simulink model "Colab_4Quad_model_01"  (R2018b)
settings: Solver=ode45  StartTime=0.0  StopTime=10  RelTol=1e-3
InitFcn:
  | Colab_4Quad_model_01_const
values from neighbouring files (symbols this model uses):
  All_rho = [d1 0 0 ... (first row only)    [Colab_4Quad_model_01_const.m]    (also in Colab_4Quad_model_02_const.m; Simple_4Quad_payload_04_const.m; Simple_4Quad_payload_05_const.m; Simple_4Quad_payload_06_const.m)
  d1 = 0.25    [Colab_4Quad_model_01_const.m]    (also in Colab_4Quad_model_02_const.m = 0.5; Simple_4Quad_payload_01_const.m = 1; Simple_4Quad_payload_02_const.m = 1; Simple_4Quad_payload_03_const.m = 1)
  d2 = 0.25    [Colab_4Quad_model_01_const.m]    (also in Colab_4Quad_model_02_const.m = 0.5; Simple_4Quad_payload_01_const.m = 1; Simple_4Quad_payload_02_const.m = 1; Simple_4Quad_payload_03_const.m = 1)
  g = 9.81    [Colab_4Quad_model_01_const.m]    (also in Colab_4Quad_model_02_const.m; Simple_2Quad_payload_01_const.m; Simple_2Quad_payload_02_const.m; Simple_2Quad_payload_03_const.m)
  Jo = diag([Ix;Iy;Iz])    [Colab_4Quad_model_01_const.m]    (also in Colab_4Quad_model_02_const.m; Simple_4Quad_payload_04_const.m; Simple_4Quad_payload_05_const.m; Simple_4Quad_payload_06_const.m)
  Jq = diag([0.0291 0.0291 0.0552])    [Colab_4Quad_model_01_const.m]    (also in Colab_4Quad_model_02_const.m = diag([0.03 0.03 0.06]); Simple_4Quad_payload_03_const.m = 1.2416e-3 * diag([1 1 2]); Simple_4Quad_payload_04_const.m = 1 * diag([1 1 2]); Simple_4Quad_payload_05_const.m = 1 * diag([1 1 2]))
  l = 3.1819    [Colab_4Quad_model_01_const.m]    (also in Colab_4Quad_model_02_const.m = 3; Simple_2Quad_payload_04_const.m = 1; Simple_4Quad_payload_01_const.m = 1; Simple_4Quad_payload_02_const.m = 2)
  M = 1.0    (= 1)    [Colab_4Quad_model_01_const.m]    (also in Colab_4Quad_model_02_const.m; Simple_2Quad_payload_01_const.m; Simple_2Quad_payload_02_const.m; Simple_2Quad_payload_03_const.m)
  m = 1.5    [Colab_4Quad_model_01_const.m]    (also in Colab_4Quad_model_02_const.m; Simple_2Quad_payload_04_const.m = 1; Simple_4Quad_payload_01_const.m = 1; Simple_4Quad_payload_02_const.m = 1)
  U0 = -20    [Colab_4Quad_model_01_const.m]    (also in Colab_4Quad_model_02_const.m)
settings Model: Creator=ali  LastModifiedBy=asafae
settings SolverCC: ZeroCrossAlgorithm=Adaptive
settings DebuggingCC: IgnoredZcDiagnostic=none

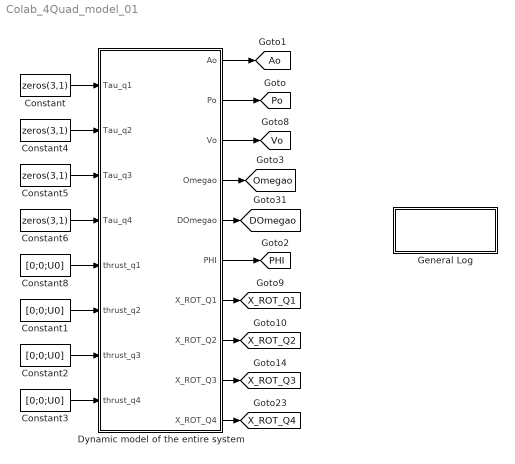
== system Colab_4Quad_model_01 ==
  Constant{,4..6} (4 alike) : Constant  Value=zeros(3,1)
  Constant{1..3,8} (4 alike) : Constant  Value=[0;0;U0]
  Dynamic model of the entire system : Subsystem
  General Log : Subsystem
  tag scope: Ao=global, DOmegao=global, Omegao=global, PHI=global, Po=global, Vo=global, X_ROT_Q1=global, X_ROT_Q2=global, X_ROT_Q3=global, X_ROT_Q4=global
  wires:
  Constant4/1 -> Dynamic model of the entire system/2(Tau_q2)
  Constant5/1 -> Dynamic model of the entire system/3(Tau_q3)
  Constant6/1 -> Dynamic model of the entire system/4(Tau_q4)
  Dynamic model of the entire system/6(PHI) -> [PHI]
  Dynamic model of the entire system/4(Omegao) -> [Omegao]
  Dynamic model of the entire system/1(Ao) -> [Ao]
  Dynamic model of the entire system/2(Po) -> [Po]
  Dynamic model of the entire system/5(DOmegao) -> [DOmegao]
  Dynamic model of the entire system/7(X_ROT_Q1) -> [X_ROT_Q1]
  Dynamic model of the entire system/8(X_ROT_Q2) -> [X_ROT_Q2]
  Dynamic model of the entire system/9(X_ROT_Q3) -> [X_ROT_Q3]
  Dynamic model of the entire system/3(Vo) -> [Vo]
  Dynamic model of the entire system/10(X_ROT_Q4) -> [X_ROT_Q4]
  Constant/1 -> Dynamic model of the entire system/1(Tau_q1)
  Constant8/1 -> Dynamic model of the entire system/5(thrust_q1)
  Constant1/1 -> Dynamic model of the entire system/6(thrust_q2)
  Constant2/1 -> Dynamic model of the entire system/7(thrust_q3)
  Constant3/1 -> Dynamic model of the entire system/8(thrust_q4)

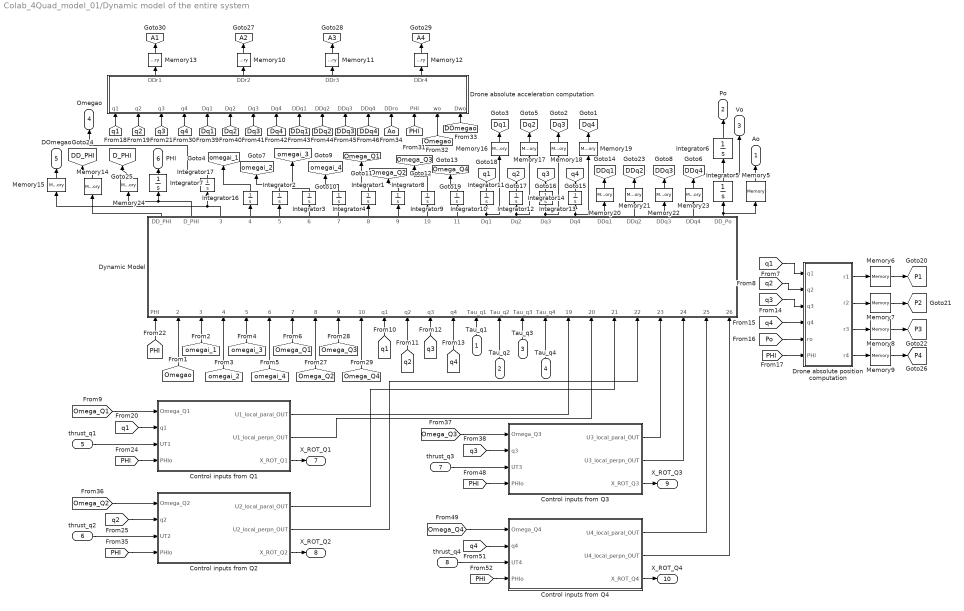
== system Colab_4Quad_model_01/Dynamic model of the entire system ==
  Tau_q1 : Inport
  Tau_q2 : Inport  Port=2
  Tau_q3 : Inport  Port=3
  Tau_q4 : Inport  Port=4
  thrust_q1 : Inport  Port=5
  thrust_q2 : Inport  Port=6
  thrust_q3 : Inport  Port=7
  thrust_q4 : Inport  Port=8
  Control inputs from Q1 : Subsystem
  Control inputs from Q2 : Subsystem
  Control inputs from Q3 : Subsystem
  Control inputs from Q4 : Subsystem
  Drone absolute acceleration computation : MATLAB Function  TreatAsAtomicUnit=on
  Drone absolute position computation : MATLAB Function  TreatAsAtomicUnit=on
  "Dynamic Model " : MATLAB Function  TreatAsAtomicUnit=on
  Integrator{1..5,7..10,16..17} (11 alike) : Integrator  InitialCondition=zeros(3,1)
  Integrator{11..14} (4 alike) : Integrator  InitialCondition=[0;0;1]
  Integrator6 : Integrator  InitialCondition=[0;0;0]
  Memory{5,10..24} (16 alike) : Memory  InitialCondition=zeros(3,1)
  Memory6 : Memory  InitialCondition=[d1;0;l]
  Memory7 : Memory  InitialCondition=[-d1;0;l]
  Memory8 : Memory  InitialCondition=[0;d2;l]
  Memory9 : Memory  InitialCondition=[0;-d2;l]
  Ao : Outport
  Po : Outport  Port=2
  Vo : Outport  Port=3
  Omegao : Outport  Port=4
  DOmegao : Outport  Port=5
  PHI : Outport  Port=6
  X_ROT_Q1 : Outport  Port=7
  X_ROT_Q2 : Outport  Port=8
  X_ROT_Q3 : Outport  Port=9
  X_ROT_Q4 : Outport  Port=10
  tag scope: A1=global, A2=global, A3=global, A4=global, DD_PHI=global, DDq1=global, DDq2=global, DDq3=global, DDq4=global, D_PHI=global, Dq1=global, Dq2=global, Dq3=global, Dq4=global, Omega_Q1=global, Omega_Q2=global, Omega_Q3=global, Omega_Q4=global, P1=global, P2=global, P3=global, P4=global, omegai_1=global, omegai_2=global, omegai_3=global, omegai_4=global, q1=global, q2=global, q3=global, q4=global
  wires:
  Integrator5/1 -> Vo/1, Integrator6/1
  Integrator1/1 -> [Omega_Q1]
  Integrator2/1 -> [omegai_2]
  Integrator3/1 -> [omegai_3]
  Integrator6/1 -> Po/1
  Integrator4/1 -> [omegai_4]
  Memory5/1 -> Ao/1
  Integrator7/1 -> PHI/1
  "Dynamic Model "/20(DD_Po) -> Memory5/1, Integrator5/1
  "Dynamic Model "/2(D_PHI) -> Memory24/1, Integrator7/1
  "Dynamic Model "/1(DD_PHI) -> Memory14/1
  "Dynamic Model "/7(D_omegai_4) -> Integrator4/1
  "Dynamic Model "/6(D_omegai_3) -> Integrator3/1
  "Dynamic Model "/5(D_omegai_2) -> Integrator2/1
  "Dynamic Model "/4(D_omegai_1) -> Integrator16/1
  "Dynamic Model "/3(D_Omegao) -> Memory15/1, Integrator17/1
  Integrator16/1 -> [omegai_1]
  "Dynamic Model "/8(D_Omega_Q1) -> Integrator1/1
  "Dynamic Model "/9(D_Omega_Q2) -> Integrator8/1
  "Dynamic Model "/10(D_Omega_Q3) -> Integrator9/1
  "Dynamic Model "/11(D_Omega_Q4) -> Integrator10/1
  Integrator8/1 -> [Omega_Q2]
  Integrator10/1 -> [Omega_Q4]
  Integrator9/1 -> [Omega_Q3]
  "Dynamic Model "/12(Dq1) -> Memory16/1, Integrator11/1
  "Dynamic Model "/13(Dq2) -> Memory17/1, Integrator12/1
  "Dynamic Model "/14(Dq3) -> Memory18/1, Integrator13/1
  "Dynamic Model "/15(Dq4) -> Memory19/1, Integrator14/1
  Integrator14/1 -> [q4]
  Integrator13/1 -> [q3]
  Integrator12/1 -> [q2]
  Integrator11/1 -> [q1]
  [PHI] -> "Dynamic Model "/1(PHI)
  [Omegao] -> "Dynamic Model "/2(Omegao)
  [omegai_1] -> "Dynamic Model "/3(omegai1)
  [omegai_2] -> "Dynamic Model "/4(omegai2)
  [omegai_3] -> "Dynamic Model "/5(omegai3)
  [omegai_4] -> "Dynamic Model "/6(omegai4)
  [Omega_Q1] -> "Dynamic Model "/7(Omega_q1)
  [Omega_Q2] -> "Dynamic Model "/8(Omega_q2)
  [Omega_Q3] -> "Dynamic Model "/9(Omega_q3)
  [Omega_Q4] -> "Dynamic Model "/10(Omega_q4)
  [q1] -> "Dynamic Model "/11(q1)
  [q2] -> "Dynamic Model "/12(q2)
  [q3] -> "Dynamic Model "/13(q3)
  [q4] -> "Dynamic Model "/14(q4)
  Tau_q2/1 -> "Dynamic Model "/16(Tau_q2)
  Tau_q4/1 -> "Dynamic Model "/18(Tau_q4)
  Tau_q1/1 -> "Dynamic Model "/15(Tau_q1)
  Tau_q3/1 -> "Dynamic Model "/17(Tau_q3)
  Control inputs from Q1/1(U1_local_paral_OUT) -> "Dynamic Model "/19(U1_local_paral)
  [q1] -> Drone absolute position computation/1(q1)
  [q2] -> Drone absolute position computation/2(q2)
  [q3] -> Drone absolute position computation/3(q3)
  [q4] -> Drone absolute position computation/4(q4)
  [Po] -> Drone absolute position computation/5(ro)
  [PHI] -> Drone absolute position computation/6(PHI)
  Memory6/1 -> [P1]
  Memory8/1 -> [P3]
  Memory7/1 -> [P2]
  Memory9/1 -> [P4]
  Drone absolute position computation/4(r4) -> Memory9/1
  Drone absolute position computation/3(r3) -> Memory8/1
  Drone absolute position computation/2(r2) -> Memory7/1
  Drone absolute position computation/1(r1) -> Memory6/1
  [q1] -> Drone absolute acceleration computation/1(q1)
  [q2] -> Drone absolute acceleration computation/2(q2)
  [q3] -> Drone absolute acceleration computation/3(q3)
  [q4] -> Drone absolute acceleration computation/4(q4)
  [PHI] -> Drone absolute acceleration computation/14(PHI)
  [Omegao] -> Drone absolute acceleration computation/15(wo)
  Memory13/1 -> [A1]
  Drone absolute acceleration computation/1(DDr1) -> Memory13/1
  Memory10/1 -> [A2]
  Drone absolute acceleration computation/2(DDr2) -> Memory10/1
  Memory11/1 -> [A3]
  Drone absolute acceleration computation/3(DDr3) -> Memory11/1
  Memory12/1 -> [A4]
  Drone absolute acceleration computation/4(DDr4) -> Memory12/1
  Memory15/1 -> DOmegao/1
  [DOmegao] -> Drone absolute acceleration computation/16(Dwo)
  [Ao] -> Drone absolute acceleration computation/13(DDro)
  Memory19/1 -> [Dq4]
  Memory18/1 -> [Dq3]
  Memory16/1 -> [Dq1]
  Memory17/1 -> [Dq2]
  [Dq4] -> Drone absolute acceleration computation/8(Dq4)
  [Dq3] -> Drone absolute acceleration computation/7(Dq3)
  [Dq2] -> Drone absolute acceleration computation/6(Dq2)
  [Dq1] -> Drone absolute acceleration computation/5(Dq1)
  Memory21/1 -> [DDq2]
  Memory20/1 -> [DDq1]
  Memory22/1 -> [DDq3]
  Memory23/1 -> [DDq4]
  "Dynamic Model "/16(DDq1) -> Memory20/1
  "Dynamic Model "/17(DDq2) -> Memory21/1
  "Dynamic Model "/18(DDq3) -> Memory22/1
  "Dynamic Model "/19(DDq4) -> Memory23/1
  [DDq1] -> Drone absolute acceleration computation/9(DDq1)
  [DDq2] -> Drone absolute acceleration computation/10(DDq2)
  [DDq3] -> Drone absolute acceleration computation/11(DDq3)
  [DDq4] -> Drone absolute acceleration computation/12(DDq4)
  Memory24/1 -> [D_PHI]
  Control inputs from Q3/1(U3_local_paral_OUT) -> "Dynamic Model "/23(U3_local_paral)
  Control inputs from Q4/1(U4_local_paral_OUT) -> "Dynamic Model "/25(U4_local_paral)
  Control inputs from Q4/2(U4_local_perpn_OUT) -> "Dynamic Model "/26(U4_local_perpn)
  Control inputs from Q1/3(X_ROT_Q1) -> X_ROT_Q1/1
  [Omega_Q1] -> Control inputs from Q1/1(Omega_Q1)
  Control inputs from Q1/2(U1_local_perpn_OUT) -> "Dynamic Model "/20(U1_local_perpn)
  [q1] -> Control inputs from Q1/2(q1)
  thrust_q1/1 -> Control inputs from Q1/3(UT1)
  [PHI] -> Control inputs from Q1/4(PHIo)
  [PHI] -> Control inputs from Q2/4(PHIo)
  thrust_q2/1 -> Control inputs from Q2/3(UT2)
  [q2] -> Control inputs from Q2/2(q2)
  [Omega_Q2] -> Control inputs from Q2/1(Omega_Q2)
  Control inputs from Q2/3(X_ROT_Q2) -> X_ROT_Q2/1
  Control inputs from Q2/1(U2_local_paral_OUT) -> "Dynamic Model "/21(U2_local_paral)
  Control inputs from Q2/2(U2_local_perpn_OUT) -> "Dynamic Model "/22(U2_local_perpn)
  [Omega_Q3] -> Control inputs from Q3/1(Omega_Q3)
  Control inputs from Q3/3(X_ROT_Q3) -> X_ROT_Q3/1
  Control inputs from Q3/2(U3_local_perpn_OUT) -> "Dynamic Model "/24(U3_local_perpn)
  [q3] -> Control inputs from Q3/2(q3)
  [PHI] -> Control inputs from Q3/4(PHIo)
  Control inputs from Q4/3(X_ROT_Q4) -> X_ROT_Q4/1
  [Omega_Q4] -> Control inputs from Q4/1(Omega_Q4)
  [q4] -> Control inputs from Q4/2(q4)
  [PHI] -> Control inputs from Q4/4(PHIo)
  Memory14/1 -> [DD_PHI]
  thrust_q4/1 -> Control inputs from Q4/3(UT4)
  Integrator17/1 -> Omegao/1
  thrust_q3/1 -> Control inputs from Q3/3(UT3)

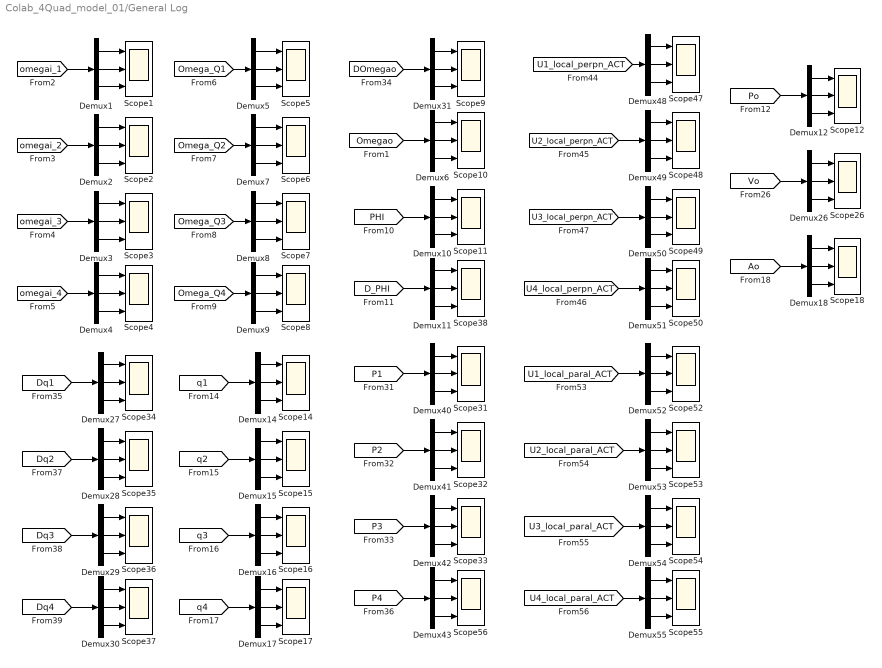
== system Colab_4Quad_model_01/General Log ==
  Demux{1..12,14..18,26..31,40..43,48..55} (35 alike) : Demux  Outputs=3
  Scope{1..12,14..18,26,31..38,47..50,52..56} (35 alike) : Scope  NumInputPorts=3
  wires:
  Demux6/2 -> Scope10/2
  Demux6/1 -> Scope10/1
  Demux6/3 -> Scope10/3
  [Omegao] -> Demux6/1
  [omegai_1] -> Demux1/1
  Demux1/3 -> Scope1/3
  Demux1/1 -> Scope1/1
  Demux1/2 -> Scope1/2
  Demux2/2 -> Scope2/2
  Demux2/1 -> Scope2/1
  Demux2/3 -> Scope2/3
  [omegai_2] -> Demux2/1
  [omegai_3] -> Demux3/1
  Demux3/3 -> Scope3/3
  Demux3/1 -> Scope3/1
  Demux3/2 -> Scope3/2
  Demux4/2 -> Scope4/2
  Demux4/1 -> Scope4/1
  Demux4/3 -> Scope4/3
  [omegai_4] -> Demux4/1
  [Omega_Q4] -> Demux9/1
  Demux9/3 -> Scope8/3
  Demux9/1 -> Scope8/1
  Demux9/2 -> Scope8/2
  Demux8/2 -> Scope7/2
  Demux8/1 -> Scope7/1
  Demux8/3 -> Scope7/3
  [Omega_Q3] -> Demux8/1
  [Omega_Q2] -> Demux7/1
  Demux7/3 -> Scope6/3
  Demux7/1 -> Scope6/1
  Demux7/2 -> Scope6/2
  Demux5/2 -> Scope5/2
  Demux5/1 -> Scope5/1
  Demux5/3 -> Scope5/3
  [Omega_Q1] -> Demux5/1
  [PHI] -> Demux10/1
  Demux10/3 -> Scope11/3
  Demux10/1 -> Scope11/1
  Demux10/2 -> Scope11/2
  Demux11/2 -> Scope38/2
  Demux11/1 -> Scope38/1
  Demux11/3 -> Scope38/3
  [D_PHI] -> Demux11/1
  [Po] -> Demux12/1
  Demux12/3 -> Scope12/3
  Demux12/1 -> Scope12/1
  Demux12/2 -> Scope12/2
  [q4] -> Demux17/1
  Demux17/3 -> Scope17/3
  Demux17/1 -> Scope17/1
  Demux17/2 -> Scope17/2
  Demux16/2 -> Scope16/2
  Demux16/1 -> Scope16/1
  Demux16/3 -> Scope16/3
  [q3] -> Demux16/1
  [q2] -> Demux15/1
  Demux15/3 -> Scope15/3
  Demux15/1 -> Scope15/1
  Demux15/2 -> Scope15/2
  Demux14/2 -> Scope14/2
  Demux14/1 -> Scope14/1
  Demux14/3 -> Scope14/3
  [q1] -> Demux14/1
  [Vo] -> Demux26/1
  Demux26/3 -> Scope26/3
  Demux26/1 -> Scope26/1
  Demux26/2 -> Scope26/2
  [DOmegao] -> Demux31/1
  Demux31/3 -> Scope9/3
  Demux31/1 -> Scope9/1
  Demux31/2 -> Scope9/2
  [Dq1] -> Demux27/1
  Demux27/3 -> Scope34/3
  Demux27/1 -> Scope34/1
  Demux27/2 -> Scope34/2
  Demux28/2 -> Scope35/2
  Demux28/1 -> Scope35/1
  Demux28/3 -> Scope35/3
  [Dq2] -> Demux28/1
  [Dq3] -> Demux29/1
  Demux29/3 -> Scope36/3
  Demux29/1 -> Scope36/1
  Demux29/2 -> Scope36/2
  Demux30/2 -> Scope37/2
  Demux30/1 -> Scope37/1
  Demux30/3 -> Scope37/3
  [Dq4] -> Demux30/1
  [P1] -> Demux40/1
  Demux40/3 -> Scope31/3
  Demux40/2 -> Scope31/2
  Demux41/2 -> Scope32/2
  Demux41/1 -> Scope32/1
  Demux41/3 -> Scope32/3
  [P2] -> Demux41/1
  [P3] -> Demux42/1
  Demux42/3 -> Scope33/3
  Demux42/1 -> Scope33/1
  Demux42/2 -> Scope33/2
  Demux43/2 -> Scope56/2
  Demux43/1 -> Scope56/1
  Demux43/3 -> Scope56/3
  [P4] -> Demux43/1
  Demux40/1 -> Scope31/1
  [U2_local_paral_ACT] -> Demux53/1
  [U3_local_paral_ACT] -> Demux54/1
  [U4_local_paral_ACT] -> Demux55/1
  [U1_local_paral_ACT] -> Demux52/1
  Demux52/3 -> Scope52/3
  Demux52/1 -> Scope52/1
  Demux52/2 -> Scope52/2
  Demux53/2 -> Scope53/2
  Demux53/1 -> Scope53/1
  Demux53/3 -> Scope53/3
  Demux54/3 -> Scope54/3
  Demux54/1 -> Scope54/1
  Demux54/2 -> Scope54/2
  Demux55/2 -> Scope55/2
  Demux55/1 -> Scope55/1
  Demux55/3 -> Scope55/3
  [U4_local_perpn_ACT] -> Demux51/1
  Demux51/3 -> Scope50/3
  Demux51/1 -> Scope50/1
  Demux51/2 -> Scope50/2
  Demux50/2 -> Scope49/2
  Demux50/1 -> Scope49/1
  Demux50/3 -> Scope49/3
  [U3_local_perpn_ACT] -> Demux50/1
  [U2_local_perpn_ACT] -> Demux49/1
  Demux49/3 -> Scope48/3
  Demux49/1 -> Scope48/1
  Demux49/2 -> Scope48/2
  Demux48/2 -> Scope47/2
  Demux48/1 -> Scope47/1
  Demux48/3 -> Scope47/3
  [U1_local_perpn_ACT] -> Demux48/1
  [Ao] -> Demux18/1
  Demux18/3 -> Scope18/3
  Demux18/1 -> Scope18/1
  Demux18/2 -> Scope18/2

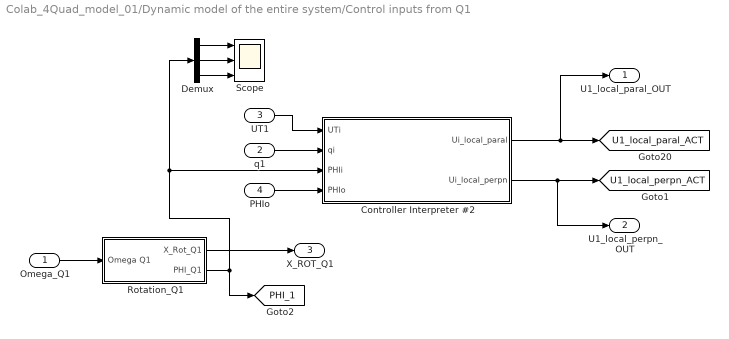
== system Colab_4Quad_model_01/Dynamic model of the entire system/Control inputs from Q1 ==
  Omega_Q1 : Inport
  q1 : Inport  Port=2
  UT1 : Inport  Port=3
  PHIo : Inport  Port=4
  Controller Interpreter #2 : MATLAB Function  TreatAsAtomicUnit=on
  Demux : Demux  Outputs=3
  Rotation_Q1 : Subsystem
  Scope : Scope  NumInputPorts=3
  U1_local_paral_OUT : Outport
  U1_local_perpn_OUT : Outport  Port=2
  X_ROT_Q1 : Outport  Port=3
  tag scope: PHI_1=global, U1_local_paral_ACT=global, U1_local_perpn_ACT=global
  wires:
  UT1/1 -> Controller Interpreter #2/1(UTi)
  q1/1 -> Controller Interpreter #2/2(qi)
  Omega_Q1/1 -> Rotation_Q1/1(Omega Q1)
  Rotation_Q1/1(X_Rot_Q1) -> X_ROT_Q1/1
  PHIo/1 -> Controller Interpreter #2/4(PHIo)
  Controller Interpreter #2/2(Ui_local_perpn) -> U1_local_perpn_OUT/1, [U1_local_perpn_ACT]
  Controller Interpreter #2/1(Ui_local_paral) -> U1_local_paral_OUT/1, [U1_local_paral_ACT]
  Demux/1 -> Scope/1
  Demux/2 -> Scope/2
  Demux/3 -> Scope/3
  Rotation_Q1/2(PHI_Q1) -> [PHI_1], Controller Interpreter #2/3(PHIi), Demux/1

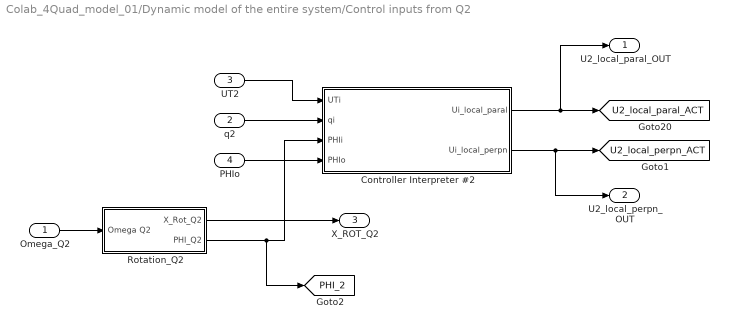
== system Colab_4Quad_model_01/Dynamic model of the entire system/Control inputs from Q2 ==
  Omega_Q2 : Inport
  q2 : Inport  Port=2
  UT2 : Inport  Port=3
  PHIo : Inport  Port=4
  Controller Interpreter #2 : MATLAB Function  TreatAsAtomicUnit=on
  Rotation_Q2 : Subsystem
  U2_local_paral_OUT : Outport
  U2_local_perpn_OUT : Outport  Port=2
  X_ROT_Q2 : Outport  Port=3
  tag scope: PHI_2=global, U2_local_paral_ACT=global, U2_local_perpn_ACT=global
  wires:
  PHIo/1 -> Controller Interpreter #2/4(PHIo)
  Rotation_Q2/1(X_Rot_Q2) -> X_ROT_Q2/1
  Omega_Q2/1 -> Rotation_Q2/1(Omega Q2)
  q2/1 -> Controller Interpreter #2/2(qi)
  UT2/1 -> Controller Interpreter #2/1(UTi)
  Controller Interpreter #2/2(Ui_local_perpn) -> U2_local_perpn_OUT/1, [U2_local_perpn_ACT]
  Controller Interpreter #2/1(Ui_local_paral) -> U2_local_paral_OUT/1, [U2_local_paral_ACT]
  Rotation_Q2/2(PHI_Q2) -> [PHI_2], Controller Interpreter #2/3(PHIi)

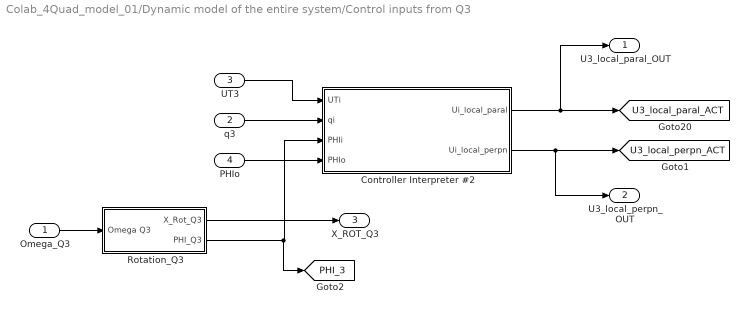
== system Colab_4Quad_model_01/Dynamic model of the entire system/Control inputs from Q3 ==
  Omega_Q3 : Inport
  q3 : Inport  Port=2
  UT3 : Inport  Port=3
  PHIo : Inport  Port=4
  Controller Interpreter #2 : MATLAB Function  TreatAsAtomicUnit=on
  Rotation_Q3 : Subsystem
  U3_local_paral_OUT : Outport
  U3_local_perpn_OUT : Outport  Port=2
  X_ROT_Q3 : Outport  Port=3
  tag scope: PHI_3=global, U3_local_paral_ACT=global, U3_local_perpn_ACT=global
  wires:
  UT3/1 -> Controller Interpreter #2/1(UTi)
  q3/1 -> Controller Interpreter #2/2(qi)
  Omega_Q3/1 -> Rotation_Q3/1(Omega Q3)
  Rotation_Q3/1(X_Rot_Q3) -> X_ROT_Q3/1
  PHIo/1 -> Controller Interpreter #2/4(PHIo)
  Controller Interpreter #2/2(Ui_local_perpn) -> U3_local_perpn_OUT/1, [U3_local_perpn_ACT]
  Controller Interpreter #2/1(Ui_local_paral) -> U3_local_paral_OUT/1, [U3_local_paral_ACT]
  Rotation_Q3/2(PHI_Q3) -> [PHI_3], Controller Interpreter #2/3(PHIi)

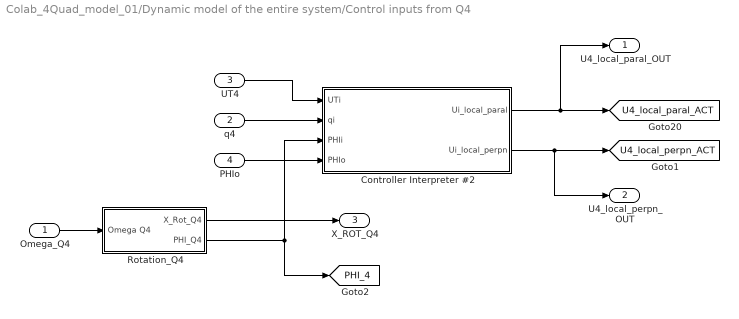
== system Colab_4Quad_model_01/Dynamic model of the entire system/Control inputs from Q4 ==
  Omega_Q4 : Inport
  q4 : Inport  Port=2
  UT4 : Inport  Port=3
  PHIo : Inport  Port=4
  Controller Interpreter #2 : MATLAB Function  TreatAsAtomicUnit=on
  Rotation_Q4 : Subsystem
  U4_local_paral_OUT : Outport
  U4_local_perpn_OUT : Outport  Port=2
  X_ROT_Q4 : Outport  Port=3
  tag scope: PHI_4=global, U4_local_paral_ACT=global, U4_local_perpn_ACT=global
  wires:
  PHIo/1 -> Controller Interpreter #2/4(PHIo)
  Rotation_Q4/1(X_Rot_Q4) -> X_ROT_Q4/1
  Omega_Q4/1 -> Rotation_Q4/1(Omega Q4)
  q4/1 -> Controller Interpreter #2/2(qi)
  UT4/1 -> Controller Interpreter #2/1(UTi)
  Controller Interpreter #2/1(Ui_local_paral) -> U4_local_paral_OUT/1, [U4_local_paral_ACT]
  Rotation_Q4/2(PHI_Q4) -> Controller Interpreter #2/3(PHIi), [PHI_4]
  Controller Interpreter #2/2(Ui_local_perpn) -> U4_local_perpn_OUT/1, [U4_local_perpn_ACT]

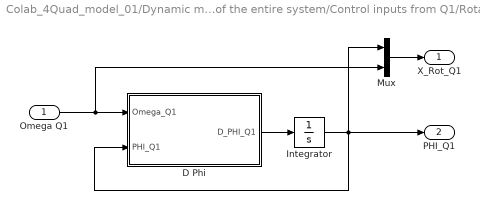
== system Colab_4Quad_model_01/Dynamic model of the entire system/Control inputs from Q1/Rotation_Q1 ==
  Omega Q1 : Inport
  D Phi : MATLAB Function  TreatAsAtomicUnit=on
  Integrator : Integrator  InitialCondition=zeros(3,1)
  Mux : Mux  Inputs=2
  X_Rot_Q1 : Outport
  PHI_Q1 : Outport  Port=2
  wires:
  D Phi/1(D_PHI_Q1) -> Integrator/1
  Omega Q1/1 -> D Phi/1(Omega_Q1), Mux/2
  Integrator/1 -> PHI_Q1/1, D Phi/2(PHI_Q1), Mux/1
  Mux/1 -> X_Rot_Q1/1

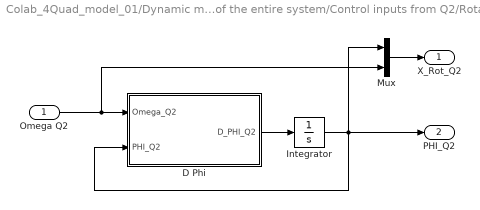
== system Colab_4Quad_model_01/Dynamic model of the entire system/Control inputs from Q2/Rotation_Q2 ==
  Omega Q2 : Inport
  D Phi : MATLAB Function  TreatAsAtomicUnit=on
  Integrator : Integrator  InitialCondition=zeros(3,1)
  Mux : Mux  Inputs=2
  X_Rot_Q2 : Outport
  PHI_Q2 : Outport  Port=2
  wires:
  D Phi/1(D_PHI_Q2) -> Integrator/1
  Omega Q2/1 -> Mux/2, D Phi/1(Omega_Q2)
  Integrator/1 -> PHI_Q2/1, D Phi/2(PHI_Q2), Mux/1
  Mux/1 -> X_Rot_Q2/1

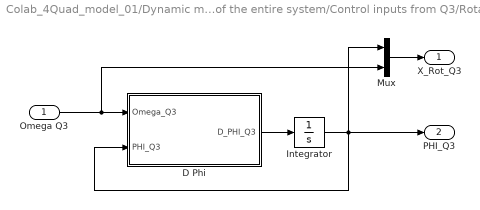
== system Colab_4Quad_model_01/Dynamic model of the entire system/Control inputs from Q3/Rotation_Q3 ==
  Omega Q3 : Inport
  D Phi : MATLAB Function  TreatAsAtomicUnit=on
  Integrator : Integrator  InitialCondition=zeros(3,1)
  Mux : Mux  Inputs=2
  X_Rot_Q3 : Outport
  PHI_Q3 : Outport  Port=2
  wires:
  D Phi/1(D_PHI_Q3) -> Integrator/1
  Omega Q3/1 -> Mux/2, D Phi/1(Omega_Q3)
  Integrator/1 -> PHI_Q3/1, D Phi/2(PHI_Q3), Mux/1
  Mux/1 -> X_Rot_Q3/1

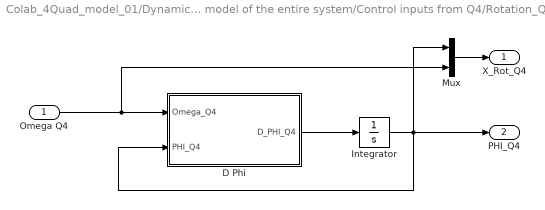
== system Colab_4Quad_model_01/Dynamic model of the entire system/Control inputs from Q4/Rotation_Q4 ==
  Omega Q4 : Inport
  D Phi : MATLAB Function  TreatAsAtomicUnit=on
  Integrator : Integrator  InitialCondition=zeros(3,1)
  Mux : Mux  Inputs=2
  X_Rot_Q4 : Outport
  PHI_Q4 : Outport  Port=2
  wires:
  D Phi/1(D_PHI_Q4) -> Integrator/1
  Integrator/1 -> PHI_Q4/1, D Phi/2(PHI_Q4), Mux/1
  Mux/1 -> X_Rot_Q4/1
  Omega Q4/1 -> D Phi/1(Omega_Q4), Mux/2

== matlab function Colab_4Quad_model_01/Dynamic model of the entire system/Control inputs from Q1/Rotation_Q1/D Phi ==
  data: Omega_Q1 input; D_PHI_Q1 output; PHI_Q1 input
function D_PHI_Q1 = fcn(Omega_Q1,PHI_Q1)

phi_q1 = PHI_Q1(1);
theta_q1 = PHI_Q1(2);

Rm_Q1 = [1 0 -sin(theta_q1);
    0 cos(phi_q1) cos(theta_q1)*sin(phi_q1);
    0 -sin(phi_q1) cos(theta_q1)*cos(phi_q1)];

D_PHI_Q1 = (Rm_Q1)^(-1) * Omega_Q1;


end

== matlab function Colab_4Quad_model_01/Dynamic model of the entire system/Dynamic Model  ==
  data: DD_PHI output; D_PHI output; D_Omegao output; D_omegai_1 output; D_omegai_2 output; D_omegai_3 output; D_omegai_4 output; D_Omega_Q1 output; D_Omega_Q2 output; D_Omega_Q3 output; D_Omega_Q4 output; Dq1 output; Dq2 output; Dq3 output; Dq4 output; DDq1 output; DDq2 output; DDq3 output; DDq4 output; PHI input; Omegao input; omegai1 input; omegai2 input; omegai3 input; omegai4 input; Omega_q1 input; Omega_q2 input; Omega_q3 input; Omega_q4 input; q1 input; q2 input; q3 input; q4 input; DD_Po output; M parameter; Jo parameter; g parameter; m parameter; l parameter; Tau_q1 input; Tau_q2 input; Tau_q3 input; Tau_q4 input; Jq parameter; U1_local_paral input; U1_local_perpn input; U2_local_paral input; U2_local_perpn input; U3_local_paral input; U3_local_perpn input; U4_local_paral input; U4_local_perpn input; All_rho parameter
function [DD_PHI,D_PHI,D_Omegao,D_omegai_1,D_omegai_2,D_omegai_3,D_omegai_4,D_Omega_Q1,D_Omega_Q2,D_Omega_Q3,D_Omega_Q4,Dq1,Dq2,Dq3,Dq4,DDq1,DDq2,DDq3,DDq4,DD_Po] = ...
    fcn(PHI,Omegao,omegai1,omegai2,omegai3,omegai4,Omega_q1,Omega_q2,Omega_q3,Omega_q4,q1,q2,q3,q4,M,Jo,g,m, l,Tau_q1,Tau_q2,Tau_q3,Tau_q4, Jq, U1_local_paral,U1_local_perpn,U2_local_paral,U2_local_perpn,...
    U3_local_paral,U3_local_perpn,U4_local_paral,U4_local_perpn, All_rho)

phi = PHI(1);
theta = PHI(2);
psi = PHI(3);

Ro = [cos(psi)*cos(theta) cos(psi)*sin(theta)*sin(phi)-sin(psi)*cos(phi) cos(psi)*sin(theta)*cos(phi)+sin(psi)*sin(phi);
    sin(psi)*cos(theta) sin(psi)*sin(theta)*sin(phi)+cos(psi)*cos(phi) sin(psi)*sin(theta)*cos(phi)-cos(psi)*sin(phi);
    -sin(theta) cos(theta)*sin(phi) cos(theta)*cos(phi)];

r1 = All_rho(1,:)';
r2 = All_rho(2,:)';
r3 = All_rho(3,:)';
r4 = All_rho(4,:)';

G = [0;0;-g];

%% 
Ui_local_paral = struct('val',repmat({zeros(3,1)},4,1));
Ui_local_perpn = struct('val',repmat({zeros(3,1)},4,1));
ri = struct('val',repmat({zeros(3,1)},4,1));
ri_skew = struct('val',repmat({zeros(3)},4,1));
qi_body = struct('val',repmat({zeros(3,1)},4,1));
qi_inert = struct('val',repmat({zeros(3,1)},4,1));
qi_inert_skew = struct('val',repmat({zeros(3)},4,1));
Mq = struct('val',repmat({zeros(3,1)},4,1));
Omega_Qi_skew = struct('val',repmat({zeros(3)},4,1));
Omega_Qi = struct('val',repmat({zeros(3,1)},4,1));
D_Omega_Qi = struct('val',repmat({zeros(3,1)},4,1));

Ui_local_paral(1).val = U1_local_paral;
Ui_local_paral(2).val = U2_local_paral;
Ui_local_paral(3).val = U3_local_paral;
Ui_local_paral(4).val = U4_local_paral;

Ui_local_perpn(1).val = U1_local_perpn;
Ui_local_perpn(2).val = U2_local_perpn;
Ui_local_perpn(3).val = U3_local_perpn;
Ui_local_perpn(4).val = U4_local_perpn;

ri(1).val = r1;
ri(2).val = r2;
ri(3).val = r3;
ri(4).val = r4;

ri_skew(1).val = ... 
    [0 -r1(3) r1(2);
    r1(3) 0 -r1(1);
    -r1(2) r1(1) 0];

ri_skew(2).val = ... 
    [0 -r2(3) r2(2);
    r2(3) 0 -r2(1);
    -r2(2) r2(1) 0];

ri_skew(3).val = ... 
    [0 -r3(3) r3(2);
    r3(3) 0 -r3(1);
    -r3(2) r3(1) 0];

ri_skew(4).val = ... 
    [0 -r4(3) r4(2);
    r4(3) 0 -r4(1);
    -r4(2) r4(1) 0];

qi_body(1).val = -[q1(1);q1(2);q1(3)];
qi_body(2).val = -[q2(1);q2(2);q2(3)];
qi_body(3).val = -[q3(1);q3(2);q3(3)];
qi_body(4).val = -[q4(1);q4(2);q4(3)];

qi_inert(1).val = Ro * qi_body(1).val;
qi_inert(2).val = Ro * qi_body(2).val;
qi_inert(3).val = Ro * qi_body(3).val;
qi_inert(4).val = Ro * qi_body(4).val;

qi_inert_skew(1).val = ...
    [0 -qi_inert(1).val(3) qi_inert(1).val(2);
    qi_inert(1).val(3) 0 -qi_inert(1).val(1);
    -qi_inert(1).val(2) qi_inert(1).val(1) 0];

qi_inert_skew(2).val = ...
    [0 -qi_inert(2).val(3) qi_inert(2).val(2);
    qi_inert(2).val(3) 0 -qi_inert(2).val(1);
    -qi_inert(2).val(2) qi_inert(2).val(1) 0];

qi_inert_skew(3).val = ...
    [0 -qi_inert(3).val(3) qi_inert(3).val(2);
    qi_inert(3).val(3) 0 -qi_inert(3).val(1);
    -qi_inert(3).val(2) qi_inert(3).val(1) 0];

qi_inert_skew(4).val = ...
    [0 -qi_inert(4).val(3) qi_inert(4).val(2);
    qi_inert(4).val(3) 0 -qi_inert(4).val(1);
    -qi_inert(4).val(2) qi_inert(4).val(1) 0];

Omegao_skew = ...
    [0 -Omegao(3) Omegao(2);
    Omegao(3) 0 -Omegao(1);
    -Omegao(2) Omegao(1) 0];

Mag2_omegai = ...
    [omegai1'*omegai1;
    omegai2'*omegai2;
    omegai3'*omegai3;
    omegai4'*omegai4];

Mq(1).val = Tau_q1;
Mq(2).val = Tau_q2;
Mq(3).val = Tau_q3;
Mq(4).val = Tau_q4;

Omega_Qi(1).val = Omega_q1;
Omega_Qi(2).val = Omega_q2;
Omega_Qi(3).val = Omega_q3;
Omega_Qi(4).val = Omega_q4;

Omega_Qi_skew(1).val = ...
    [0 -Omega_Qi(1).val(3) Omega_Qi(1).val(2);
    Omega_Qi(1).val(3) 0 -Omega_Qi(1).val(1);
    -Omega_Qi(1).val(2) Omega_Qi(1).val(1) 0];

Omega_Qi_skew(2).val = ...
    [0 -Omega_Qi(2).val(3) Omega_Qi(2).val(2);
    Omega_Qi(2).val(3) 0 -Omega_Qi(2).val(1);
    -Omega_Qi(2).val(2) Omega_Qi(2).val(1) 0];

Omega_Qi_skew(3).val = ...
    [0 -Omega_Qi(3).val(3) Omega_Qi(3).val(2);
    Omega_Qi(3).val(3) 0 -Omega_Qi(3).val(1);
    -Omega_Qi(3).val(2) Omega_Qi(3).val(1) 0];

Omega_Qi_skew(4).val = ...
    [0 -Omega_Qi(4).val(3) Omega_Qi(4).val(2);
    Omega_Qi(4).val(3) 0 -Omega_Qi(4).val(1);
    -Omega_Qi(4).val(2) Omega_Qi(4).val(1) 0];


%% Dynamics of the entire system
u_DDP = zeros(3,1);
u_DOmega = zeros(3,1);
term_g_DDP = M*eye(3)*G;
term_DOmega_DDP = zeros(3);
term_Omega2_DDP = zeros(3,1);
term_omegai2_DDP = zeros(3,1);
term_DOmega_DOmega = zeros(3);
term_Omega2_DOmega = zeros(3,1);
term_DDP_DOmega = zeros(3);
term_omegai2_DOmega = zeros(3,1);
term_g_DOmega = zeros(3,1);

M_tot = zeros(18,18);
M_tot(1:3,1:3) = M * eye(3);
F_tot = zeros(18,1);

for i=1:4
    u_DDP = u_DDP + ( Ro * Ui_local_paral(i).val ); 
    u_DOmega = u_DOmega + ( ri_skew(i).val * Ui_local_paral(i).val ); 
    term_DOmega_DDP = term_DOmega_DDP + ( m * eye(3) * Ro * ri_skew(i).val ); %qi_inert(i).val * qi_inert(i).val'
    term_Omega2_DDP = term_Omega2_DDP + ( m * eye(3) * Ro * Omegao_skew * Omegao_skew * ri(i).val ); %qi_inert(i).val * qi_inert(i).val'
    term_omegai2_DDP = term_omegai2_DDP + ( m * l * Mag2_omegai(i) * qi_inert(i).val );
    term_DOmega_DOmega = term_DOmega_DOmega + ( m * ri_skew(i).val * Ro' * eye(3) * Ro * ri_skew(i).val ); %qi_inert(i).val * qi_inert(i).val'
    term_Omega2_DOmega = term_Omega2_DOmega + ( m * ri_skew(i).val * Ro' * eye(3) * Ro * Omegao_skew * Omegao_skew * ri(i).val ); %qi_inert(i).val * qi_inert(i).val'
    term_omegai2_DOmega = term_omegai2_DOmega + ( m * l * ri_skew(i).val * Ro' * Mag2_omegai(i) * qi_inert(i).val );
    term_DDP_DOmega = term_DDP_DOmega + ( m * ri_skew(i).val * Ro' * eye(3) ); %qi_inert(i).val * qi_inert(i).val'
    term_g_DOmega = term_g_DOmega + ( m * ri_skew(i).val * Ro' * eye(3) * G ); %qi_inert(i).val * qi_inert(i).val'
    term_g_DDP = term_g_DDP + ( m * eye(3) * G); %qi_inert(i).val * qi_inert(i).val'
    
    M_tot(1:3,1:3) = M_tot(1:3,1:3) + ( m * eye(3) ); %qi_inert(i).val * qi_inert(i).val'
    
    M_tot(6+(i-1)*3+1:6+(i-1)*3+3,1:3) = -m * qi_inert_skew(i).val; 
    M_tot(6+(i-1)*3+1:6+(i-1)*3+3,4:6) = m * qi_inert_skew(i).val * Ro * ri_skew(i).val; 
    M_tot(6+(i-1)*3+1:6+(i-1)*3+3,6+(i-1)*3+1:6+(i-1)*3+3) = m * l * eye(3);
    
    F_tot(6+(i-1)*3+1:6+(i-1)*3+3,1) = qi_inert_skew(i).val * ( ( m * G ) + ( m * Ro * Omegao_skew * Omegao_skew * ri(i).val ) - ( Ro * Ui_local_perpn(i).val ) ); 
    
    D_Omega_Qi(i).val = (Jq ^ (-1)) * ( Mq(i).val - (Omega_Qi_skew(i).val * Jq * Omega_Qi(i).val) );
end

M_tot(1:3,4:6) = -1 * term_DOmega_DDP;

M_tot(4:6,1:3) = term_DDP_DOmega;
M_tot(4:6,4:6) = Jo - term_DOmega_DOmega;

F_tot(1:3,1) = u_DDP + term_g_DDP - term_omegai2_DDP - term_Omega2_DDP;
F_tot(4:6,1) = u_DOmega - term_g_DOmega - (Omegao_skew * Jo * Omegao) - term_omegai2_DOmega - term_Omega2_DOmega;

DX_tot = M_tot^(-1) * F_tot;

DD_Po = DX_tot(1:3,1);
D_Omegao = DX_tot(4:6,1);
D_omegai_1 = DX_tot(7:9,1);
D_omegai_2 = DX_tot(10:12,1);
D_omegai_3 = DX_tot(13:15,1);
D_omegai_4 = DX_tot(16:18,1);

D_Omega_Q1 = D_Omega_Qi(1).val;
D_Omega_Q2 = D_Omega_Qi(2).val;
D_Omega_Q3 = D_Omega_Qi(3).val;
D_Omega_Q4 = D_Omega_Qi(4).val;

%% Angles of links and their rates
omega1_skew = ...
    [0 -omegai1(3) omegai1(2);
    omegai1(3) 0 -omegai1(1);
    -omegai1(2) omegai1(1) 0];

omega2_skew = ...
    [0 -omegai2(3) omegai2(2);
    omegai2(3) 0 -omegai2(1);
    -omegai2(2) omegai2(1) 0];

omega3_skew = ...
    [0 -omegai3(3) omegai3(2);
    omegai3(3) 0 -omegai3(1);
    -omegai3(2) omegai3(1) 0];

omega4_skew = ...
    [0 -omegai4(3) omegai4(2);
    omegai4(3) 0 -omegai4(1);
    -omegai4(2) omegai4(1) 0];

Dq1_inert = omega1_skew * qi_inert(1).val; 
Dq2_inert = omega2_skew * qi_inert(2).val; 
Dq3_inert = omega3_skew * qi_inert(3).val; 
Dq4_inert = omega4_skew * qi_inert(4).val; 

Dq1 = Ro' * -[Dq1_inert(1);Dq1_inert(2);Dq1_inert(3)];
Dq2 = Ro' * -[Dq2_inert(1);Dq2_inert(2);Dq2_inert(3)];
Dq3 = Ro' * -[Dq3_inert(1);Dq3_inert(2);Dq3_inert(3)];
Dq4 = Ro' * -[Dq4_inert(1);Dq4_inert(2);Dq4_inert(3)];

Domega1_skew = ...
    [0 -D_omegai_1(3) D_omegai_1(2);
    D_omegai_1(3) 0 -D_omegai_1(1);
    -D_omegai_1(2) D_omegai_1(1) 0];

Domega2_skew = ...
    [0 -D_omegai_2(3) D_omegai_2(2);
    D_omegai_2(3) 0 -D_omegai_2(1);
    -D_omegai_2(2) D_omegai_2(1) 0];

Domega3_skew = ...
    [0 -D_omegai_3(3) D_omegai_3(2);
    D_omegai_3(3) 0 -D_omegai_3(1);
    -D_omegai_3(2) D_omegai_3(1) 0];

Domega4_skew = ...
    [0 -D_omegai_4(3) D_omegai_4(2);
    D_omegai_4(3) 0 -D_omegai_4(1);
    -D_omegai_4(2) D_omegai_4(1) 0];

DDq1_inert = Domega1_skew*qi_inert(1).val + omega1_skew*Dq1_inert;
DDq2_inert = Domega2_skew*qi_inert(2).val + omega2_skew*Dq2_inert;
DDq3_inert = Domega3_skew*qi_inert(3).val + omega3_skew*Dq3_inert;
DDq4_inert = Domega4_skew*qi_inert(4).val + omega4_skew*Dq4_inert;

DDq1 = Ro' * [-DDq1_inert(1);-DDq1_inert(2);-DDq1_inert(3)];
DDq2 = Ro' * [-DDq2_inert(1);-DDq2_inert(2);-DDq2_inert(3)];
DDq3 = Ro' * [-DDq3_inert(1);-DDq3_inert(2);-DDq3_inert(3)];
DDq4 = Ro' * [-DDq4_inert(1);-DDq4_inert(2);-DDq4_inert(3)];

%% Euler angles of the payload and their rates
R_f_o = [1 0 -sin(theta);
    0 cos(phi) cos(theta)*sin(phi);
    0 -sin(phi) cos(theta)*cos(phi)];

D_PHI = (R_f_o^-1) * Omegao;

DR_f_o = [0 0 -D_PHI(2)*cos(theta);
    0 -D_PHI(1)*sin(phi) (-D_PHI(2)*sin(theta)*sin(phi))+(D_PHI(1)*cos(theta)*cos(phi));
    0 -D_PHI(1)*cos(phi) (-D_PHI(2)*sin(theta)*cos(phi))-(D_PHI(1)*cos(theta)*sin(phi))];

DD_PHI = (R_f_o^-1) * ( D_Omegao - DR_f_o*D_PHI );

end

== matlab function Colab_4Quad_model_01/Dynamic model of the entire system/Control inputs from Q2/Rotation_Q2/D Phi ==
  data: Omega_Q2 input; D_PHI_Q2 output; PHI_Q2 input
function D_PHI_Q2 = fcn(Omega_Q2,PHI_Q2)

phi_q2 = PHI_Q2(1);
theta_q2 = PHI_Q2(2);

Rm_Q2 = [1 0 -sin(theta_q2);
    0 cos(phi_q2) cos(theta_q2)*sin(phi_q2);
    0 -sin(phi_q2) cos(theta_q2)*cos(phi_q2)];

D_PHI_Q2 = (Rm_Q2)^(-1) * Omega_Q2;


end

== matlab function Colab_4Quad_model_01/Dynamic model of the entire system/Control inputs from Q3/Rotation_Q3/D Phi ==
  data: Omega_Q3 input; D_PHI_Q3 output; PHI_Q3 input
function D_PHI_Q3 = fcn(Omega_Q3,PHI_Q3)

phi_q3 = PHI_Q3(1);
theta_q3 = PHI_Q3(2);

Rm_Q3 = [1 0 -sin(theta_q3);
    0 cos(phi_q3) cos(theta_q3)*sin(phi_q3);
    0 -sin(phi_q3) cos(theta_q3)*cos(phi_q3)];

D_PHI_Q3 = (Rm_Q3)^(-1) * Omega_Q3;


end

== matlab function Colab_4Quad_model_01/Dynamic model of the entire system/Control inputs from Q4/Rotation_Q4/D Phi ==
  data: Omega_Q4 input; D_PHI_Q4 output; PHI_Q4 input
function D_PHI_Q4 = fcn(Omega_Q4,PHI_Q4)

phi_q4 = PHI_Q4(1);
theta_q4 = PHI_Q4(2);

Rm_Q4 = [1 0 -sin(theta_q4);
    0 cos(phi_q4) cos(theta_q4)*sin(phi_q4);
    0 -sin(phi_q4) cos(theta_q4)*cos(phi_q4)];

D_PHI_Q4 = (Rm_Q4)^(-1) * Omega_Q4;

end

== matlab function Colab_4Quad_model_01/Dynamic model of the entire system/Drone absolute position computation ==
  data: q1 input; r1 output; r2 output; r3 output; r4 output; q2 input; q3 input; q4 input; All_rho parameter; l parameter; ro input; PHI input
function [r1,r2,r3,r4] = fcn(q1,q2,q3,q4,All_rho, l,ro,PHI)

rho1 = All_rho(1,:)';
rho2 = All_rho(2,:)';
rho3 = All_rho(3,:)';
rho4 = All_rho(4,:)';

phi = PHI(1);
theta = PHI(2);
psi = PHI(3);

Ro = [cos(psi)*cos(theta) cos(psi)*sin(theta)*sin(phi)-sin(psi)*cos(phi) cos(psi)*sin(theta)*cos(phi)+sin(psi)*sin(phi);
    sin(psi)*cos(theta) sin(psi)*sin(theta)*sin(phi)+cos(psi)*cos(phi) sin(psi)*sin(theta)*cos(phi)-cos(psi)*sin(phi);
    -sin(theta) cos(theta)*sin(phi) cos(theta)*cos(phi)];

r1 = ro + Ro*rho1 + l*Ro*q1;
r2 = ro + Ro*rho2 + l*Ro*q2;
r3 = ro + Ro*rho3 + l*Ro*q3;
r4 = ro + Ro*rho4 + l*Ro*q4;

end

== matlab function Colab_4Quad_model_01/Dynamic model of the entire system/Drone absolute acceleration computation ==
  data: q1 input; DDr1 output; DDr2 output; DDr3 output; DDr4 output; q2 input; q3 input; q4 input; Dq1 input; Dq2 input; Dq3 input; Dq4 input; DDq1 input; DDq2 input; DDq3 input; DDq4 input; All_rho parameter; l parameter; DDro input; PHI input; wo input; Dwo input
function [DDr1,DDr2,DDr3,DDr4] = fcn(q1,q2,q3,q4,Dq1,Dq2,Dq3,Dq4,DDq1,DDq2,DDq3,DDq4,All_rho, l,DDro,PHI,wo,Dwo)

rho1 = All_rho(1,:)';
rho2 = All_rho(2,:)';
rho3 = All_rho(3,:)';
rho4 = All_rho(4,:)';

phi = PHI(1);
theta = PHI(2);
psi = PHI(3);

wo_skew = [...
    0 -wo(3) wo(2);
    wo(3) 0 -wo(1);
    -wo(2) wo(1) 0];

Dwo_skew = [...
    0 -Dwo(3) Dwo(2);
    Dwo(3) 0 -Dwo(1);
    -Dwo(2) Dwo(1) 0];

Ro = [cos(psi)*cos(theta) cos(psi)*sin(theta)*sin(phi)-sin(psi)*cos(phi) cos(psi)*sin(theta)*cos(phi)+sin(psi)*sin(phi);
    sin(psi)*cos(theta) sin(psi)*sin(theta)*sin(phi)+cos(psi)*cos(phi) sin(psi)*sin(theta)*cos(phi)-cos(psi)*sin(phi);
    -sin(theta) cos(theta)*sin(phi) cos(theta)*cos(phi)];

DDr1 = DDro + Ro*wo_skew*wo_skew*rho1 + Ro*Dwo_skew*rho1 + l*Ro*wo_skew*wo_skew*q1 + l*Ro*Dwo_skew*q1 + 2*l*Ro*wo_skew*Dq1 + l*Ro*DDq1;
DDr2 = DDro + Ro*wo_skew*wo_skew*rho2 + Ro*Dwo_skew*rho2 + l*Ro*wo_skew*wo_skew*q2 + l*Ro*Dwo_skew*q2 + 2*l*Ro*wo_skew*Dq2 + l*Ro*DDq2;
DDr3 = DDro + Ro*wo_skew*wo_skew*rho3 + Ro*Dwo_skew*rho3 + l*Ro*wo_skew*wo_skew*q3 + l*Ro*Dwo_skew*q3 + 2*l*Ro*wo_skew*Dq3 + l*Ro*DDq3;
DDr4 = DDro + Ro*wo_skew*wo_skew*rho4 + Ro*Dwo_skew*rho4 + l*Ro*wo_skew*wo_skew*q4 + l*Ro*Dwo_skew*q4 + 2*l*Ro*wo_skew*Dq4 + l*Ro*DDq4;


end

== matlab function Colab_4Quad_model_01/Dynamic model of the entire system/Control inputs from Q1/Controller Interpreter #2 ==
  data: UTi input; qi input; PHIi input; Ui_local_paral output; PHIo input; Ui_local_perpn output
function [Ui_local_paral,Ui_local_perpn] = fcn(UTi,qi,PHIi,PHIo)

phi_i = PHIi(1);
theta_i = PHIi(2);
psi_i = PHIi(3);

Ri = [cos(psi_i)*cos(theta_i) cos(psi_i)*sin(theta_i)*sin(phi_i)-sin(psi_i)*cos(phi_i) cos(psi_i)*sin(theta_i)*cos(phi_i)+sin(psi_i)*sin(phi_i);
    sin(psi_i)*cos(theta_i) sin(psi_i)*sin(theta_i)*sin(phi_i)+cos(psi_i)*cos(phi_i) sin(psi_i)*sin(theta_i)*cos(phi_i)-cos(psi_i)*sin(phi_i);
    -sin(theta_i) cos(theta_i)*sin(phi_i) cos(theta_i)*cos(phi_i)]; 

phio = PHIo(1);
thetao = PHIo(2);
psio = PHIo(3);

Ro = [cos(psio)*cos(thetao) cos(psio)*sin(thetao)*sin(phio)-sin(psio)*cos(phio) cos(psio)*sin(thetao)*cos(phio)+sin(psio)*sin(phio);
    sin(psio)*cos(thetao) sin(psio)*sin(thetao)*sin(phio)+cos(psio)*cos(phio) sin(psio)*sin(thetao)*cos(phio)-cos(psio)*sin(phio);
    -sin(thetao) cos(thetao)*sin(phio) cos(thetao)*cos(phio)];

Ui_local_paral = (qi*qi') * (Ro' * Ri * UTi);
Ui_local_perpn = (eye(3) - qi*qi') * (Ro' * Ri * UTi);


end

== matlab function Colab_4Quad_model_01/Dynamic model of the entire system/Control inputs from Q2/Controller Interpreter #2 ==
  data: UTi input; qi input; PHIi input; Ui_local_paral output; PHIo input; Ui_local_perpn output
function [Ui_local_paral,Ui_local_perpn] = fcn(UTi,qi,PHIi,PHIo)

phi_i = PHIi(1);
theta_i = PHIi(2);
psi_i = PHIi(3);

Ri = [cos(psi_i)*cos(theta_i) cos(psi_i)*sin(theta_i)*sin(phi_i)-sin(psi_i)*cos(phi_i) cos(psi_i)*sin(theta_i)*cos(phi_i)+sin(psi_i)*sin(phi_i);
    sin(psi_i)*cos(theta_i) sin(psi_i)*sin(theta_i)*sin(phi_i)+cos(psi_i)*cos(phi_i) sin(psi_i)*sin(theta_i)*cos(phi_i)-cos(psi_i)*sin(phi_i);
    -sin(theta_i) cos(theta_i)*sin(phi_i) cos(theta_i)*cos(phi_i)]; 

phio = PHIo(1);
thetao = PHIo(2);
psio = PHIo(3);

Ro = [cos(psio)*cos(thetao) cos(psio)*sin(thetao)*sin(phio)-sin(psio)*cos(phio) cos(psio)*sin(thetao)*cos(phio)+sin(psio)*sin(phio);
    sin(psio)*cos(thetao) sin(psio)*sin(thetao)*sin(phio)+cos(psio)*cos(phio) sin(psio)*sin(thetao)*cos(phio)-cos(psio)*sin(phio);
    -sin(thetao) cos(thetao)*sin(phio) cos(thetao)*cos(phio)];

Ui_local_paral = (qi*qi') * (Ro' * Ri * UTi);
Ui_local_perpn = (eye(3) - qi*qi') * (Ro' * Ri * UTi);


end

== matlab function Colab_4Quad_model_01/Dynamic model of the entire system/Control inputs from Q3/Controller Interpreter #2 ==
  data: UTi input; qi input; PHIi input; Ui_local_paral output; PHIo input; Ui_local_perpn output
function [Ui_local_paral,Ui_local_perpn] = fcn(UTi,qi,PHIi,PHIo)

phi_i = PHIi(1);
theta_i = PHIi(2);
psi_i = PHIi(3);

Ri = [cos(psi_i)*cos(theta_i) cos(psi_i)*sin(theta_i)*sin(phi_i)-sin(psi_i)*cos(phi_i) cos(psi_i)*sin(theta_i)*cos(phi_i)+sin(psi_i)*sin(phi_i);
    sin(psi_i)*cos(theta_i) sin(psi_i)*sin(theta_i)*sin(phi_i)+cos(psi_i)*cos(phi_i) sin(psi_i)*sin(theta_i)*cos(phi_i)-cos(psi_i)*sin(phi_i);
    -sin(theta_i) cos(theta_i)*sin(phi_i) cos(theta_i)*cos(phi_i)]; 

phio = PHIo(1);
thetao = PHIo(2);
psio = PHIo(3);

Ro = [cos(psio)*cos(thetao) cos(psio)*sin(thetao)*sin(phio)-sin(psio)*cos(phio) cos(psio)*sin(thetao)*cos(phio)+sin(psio)*sin(phio);
    sin(psio)*cos(thetao) sin(psio)*sin(thetao)*sin(phio)+cos(psio)*cos(phio) sin(psio)*sin(thetao)*cos(phio)-cos(psio)*sin(phio);
    -sin(thetao) cos(thetao)*sin(phio) cos(thetao)*cos(phio)];

Ui_local_paral = (qi*qi') * (Ro' * Ri * UTi);
Ui_local_perpn = (eye(3) - qi*qi') * (Ro' * Ri * UTi);


end

== matlab function Colab_4Quad_model_01/Dynamic model of the entire system/Control inputs from Q4/Controller Interpreter #2 ==
  data: UTi input; qi input; PHIi input; Ui_local_paral output; PHIo input; Ui_local_perpn output
function [Ui_local_paral,Ui_local_perpn] = fcn(UTi,qi,PHIi,PHIo)

phi_i = PHIi(1);
theta_i = PHIi(2);
psi_i = PHIi(3);

Ri = [cos(psi_i)*cos(theta_i) cos(psi_i)*sin(theta_i)*sin(phi_i)-sin(psi_i)*cos(phi_i) cos(psi_i)*sin(theta_i)*cos(phi_i)+sin(psi_i)*sin(phi_i);
    sin(psi_i)*cos(theta_i) sin(psi_i)*sin(theta_i)*sin(phi_i)+cos(psi_i)*cos(phi_i) sin(psi_i)*sin(theta_i)*cos(phi_i)-cos(psi_i)*sin(phi_i);
    -sin(theta_i) cos(theta_i)*sin(phi_i) cos(theta_i)*cos(phi_i)]; 

phio = PHIo(1);
thetao = PHIo(2);
psio = PHIo(3);

Ro = [cos(psio)*cos(thetao) cos(psio)*sin(thetao)*sin(phio)-sin(psio)*cos(phio) cos(psio)*sin(thetao)*cos(phio)+sin(psio)*sin(phio);
    sin(psio)*cos(thetao) sin(psio)*sin(thetao)*sin(phio)+cos(psio)*cos(phio) sin(psio)*sin(thetao)*cos(phio)-cos(psio)*sin(phio);
    -sin(thetao) cos(thetao)*sin(phio) cos(thetao)*cos(phio)];

Ui_local_paral = (qi*qi') * (Ro' * Ri * UTi);
Ui_local_perpn = (eye(3) - qi*qi') * (Ro' * Ri * UTi);


end
